simulink model "soc_WLAN_fpga"  (R2024b)
settings: Solver=FixedStepDiscrete  StartTime=0.0  StopTime=stopTime  RelTol=1e-3
PreLoadFcn:
  | addpath(fullfile(matlabroot,'toolbox','whdl','whdlexamples','whdlexamples'));
InitFcn:
  | addpath(fullfile(matlabroot,'toolbox','whdl','whdlexamples','whdlexamples'));
model workspace (MAT data in the model file):
  socvcb : containers.Map (value not decoded)
undefined symbols (not defined in the file): Add, bitRatePerOfdmSym, chanBW, coe, cpLen, dataUpsampleFactor, DelayValMaxNsdMinusLastPilotSc, DescramblerInitialSeed, designMultirateFIR, fftLen, filterLatency, filterUpsampleFactor, Fs, Hd, HT_MFMCS0, HT_MFMCS1, HT_MFMCS2, HT_MFMCS3, HT_MFMCS4, HT_MFMCS5, HT_MFMCS6, HT_MFMCS7, HTUnUsedScInd, inputSamplingRate, interp_coeff, maxPilotRefCounterVale, maxPilotsRef, maxPilotsRefNonHT, Ncol_HT, Ncol_NonHT, noDataSubCarriers, Non_HTMCS0, Non_HTMCS1, Non_HTMCS2, Non_HTMCS3, Non_HTMCS4, Non_HTMCS5, Non_HTMCS6, Non_HTMCS7, Nrow_HT, Nrow_NonHT, numDSC_HT, numDSC_HT_vhtSigB, numDSC_NonHT, numDscHT, numDscNonHT, numOfBitsPerOFDMSym, numOfDataBitsPerOFDMSym, numPilots, numScHT, numSCS_HT, numSCS_NonHT, pnSeq, QAM, rxDownsampleFactor, secondPIdx_HT, secondPIdx_NonHT, Shift, VHTMCS0, VHTMCS1 ... (+7)
libraries: hdlsllib x267, simulink x210, dspsigops x22, whdlutilities x10, whdlmod x9, dsphdlfiltering2 x5, dsphdlmathfun2 x4, whdledac x3, hwlogicconnlib x2, commhdlcrc x2, dsphdlsigops2 x2
(part 3 of 14)

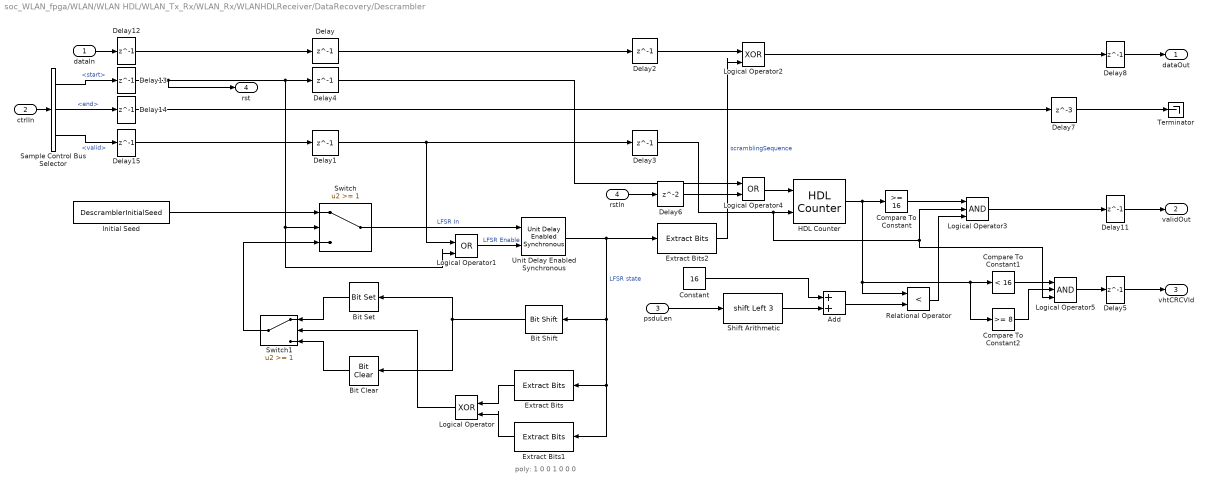
== system soc_WLAN_fpga/WLAN/WLAN HDL/WLAN_Tx_Rx/WLAN_Rx/WLANHDLReceiver/DataRecovery/Descrambler ==
  note: poly: 1 0 0 1 0 0 0
  dataIn : Inport
  ctrlIn : Inport  Port=2
  psduLen : Inport  Port=3
  rstIn : Inport  Port=4
  Add : Sum
  Bit Clear : simulink/Logic and Bit Operations/Bit Clear  iBit=0
  Bit Set : simulink/Logic and Bit Operations/Bit Set  iBit=0
  Bit Shift : hdlsllib/Logic and Bit Operations/Bit Shift  mode=Shift Left Logical  N=1
  Compare To Constant : simulink/Logic and Bit Operations/Compare To Constant  relop=>=  const=16  OutDataTypeStr=boolean
  Compare To Constant1 : simulink/Logic and Bit Operations/Compare To Constant  relop=<  const=16  OutDataTypeStr=boolean
  Compare To Constant2 : simulink/Logic and Bit Operations/Compare To Constant  relop=>=  const=8  OutDataTypeStr=boolean
  Constant : Constant  Value=16  OutDataTypeStr=fixdt(0,5,0)  SampleTime=-1
  Delay{,1..4} (5 alike) : Delay  DelayLength=1
  Delay{5,8,11..15} (7 alike) : Delay  DelayLength=1  InitialCondition=0
  Delay6 : Delay
  Delay7 : Delay  DelayLength=3
  Extract Bits : simulink/Logic and Bit Operations/Extract Bits  bitsToExtract=Range of bits  numBits=8  bitIdxRange=3  outScalingMode=Preserve fixed-point scaling
  Extract Bits1 : simulink/Logic and Bit Operations/Extract Bits  bitsToExtract=Range of bits  numBits=8  bitIdxRange=6  outScalingMode=Preserve fixed-point scaling
  Extract Bits2 : simulink/Logic and Bit Operations/Extract Bits  bitsToExtract=Range of bits  numBits=8  bitIdxRange=0  outScalingMode=Preserve fixed-point scaling
  HDL Counter : hdlsllib/Sources/HDL Counter  CountType=Count limited  CountInit=0  CountStep=1  CountMax=2^32-1  CountFromType=Initial value  CountFrom=0  CountResetPort=on  CountLoadPort=off  CountEnbPort=on  CountDirPort=off  CountHitOutputPort=off  CountDataType=Unsigned  CountWordLen=32  CountFracLen=0  CountSampTime=1
  Initial Seed : Constant  Value=DescramblerInitialSeed  OutDataTypeStr=fixdt(0,7,0)  SampleTime=-1
  Logical Operator : Logic  Operator=XOR  IconShape=distinctive  AllPortsSameDT=off  OutDataTypeStr=boolean
  Logical Operator1 : Logic  Operator=OR  IconShape=distinctive  AllPortsSameDT=off  OutDataTypeStr=boolean
  Logical Operator2 : Logic  Operator=XOR  IconShape=distinctive  AllPortsSameDT=off  OutDataTypeStr=boolean
  Logical Operator3 : Logic  Inputs=3  AllPortsSameDT=off  OutDataTypeStr=boolean
  Logical Operator4 : Logic  Operator=OR  AllPortsSameDT=off  OutDataTypeStr=boolean
  Logical Operator5 : Logic  Inputs=3  AllPortsSameDT=off  OutDataTypeStr=boolean
  Relational Operator : RelationalOperator  Operator=<  OutDataTypeStr=boolean  RndMeth=Simplest  InputSameDT=off
  Sample Control Bus Selector : whdlutilities/Sample Control Bus Selector  OutputSignals=start,end,valid
  Shift Arithmetic : ArithShift  BitShiftNumber=3  BitShiftDirection=Left
  Switch : Switch  Threshold=1  SaturateOnIntegerOverflow=off  InputSameDT=off
  Switch1 : Switch  Threshold=1  SaturateOnIntegerOverflow=off  InputSameDT=off
  Terminator : Terminator
  Unit Delay Enabled Synchronous : hdlsllib/Discrete/Unit Delay Enabled Synchronous  InitialCondition=0.0  SampleTime=-1
  dataOut : Outport
  validOut : Outport  Port=2
  vhtCRCVld : Outport  Port=3
  rst : Outport  Port=4
  wires:
  Delay15/1 -> Delay1/1
  Delay13/1 -> rst/1, Delay4/1, Switch/2, Logical Operator1/2
  Delay12/1 -> Delay/1
  Delay8/1 -> dataOut/1
  Delay4/1 -> Logical Operator4/1
  Delay2/1 -> Logical Operator2/1
  Logical Operator2/1 -> Delay8/1
  Delay1/1 -> Delay3/1, Logical Operator1/1
  Delay/1 -> Delay2/1
  Logical Operator1/1 -> Unit Delay Enabled Synchronous/2  "LFSR Enable"
  Switch1/1 -> Switch/3
  Bit Shift/1 -> Bit Set/1, Bit Clear/1
  Logical Operator/1 -> Switch1/2
  Bit Clear/1 -> Switch1/3
  Bit Set/1 -> Switch1/1
  Extract Bits1/1 -> Logical Operator/2
  Extract Bits/1 -> Logical Operator/1
  Extract Bits2/1 -> Logical Operator2/2  "scramblingSequence"
  dataIn/1 -> Delay12/1
  Unit Delay Enabled Synchronous/1 -> Extract Bits2/1, Extract Bits/1, Extract Bits1/1, Bit Shift/1  "LFSR state"
  Initial Seed/1 -> Switch/1
  Switch/1 -> Unit Delay Enabled Synchronous/1  "LFSR In"
  ctrlIn/1 -> Sample Control Bus Selector/1
  HDL Counter/1 -> Compare To Constant/1, Compare To Constant2/1, Compare To Constant1/1, Relational Operator/1
  Compare To Constant/1 -> Logical Operator3/1
  Shift Arithmetic/1 -> Add/2
  Constant/1 -> Add/1
  Relational Operator/1 -> Logical Operator3/3
  Logical Operator4/1 -> HDL Counter/1
  rstIn/1 -> Delay6/1
  Delay6/1 -> Logical Operator4/2
  Sample Control Bus Selector/1 -> Delay13/1  "<start>"
  Sample Control Bus Selector/2 -> Delay14/1  "<end>"
  Sample Control Bus Selector/3 -> Delay15/1  "<valid>"
  Delay11/1 -> validOut/1
  Compare To Constant1/1 -> Logical Operator5/1
  Compare To Constant2/1 -> Logical Operator5/2
  Delay5/1 -> vhtCRCVld/1
  Delay7/1 -> Terminator/1
  Delay14/1 -> Delay7/1
  Delay3/1 -> Logical Operator5/3, Logical Operator3/2, HDL Counter/2
  Add/1 -> Relational Operator/2
  Logical Operator3/1 -> Delay11/1
  Logical Operator5/1 -> Delay5/1
  psduLen/1 -> Shift Arithmetic/1

== system soc_WLAN_fpga/WLAN/WLAN HDL/WLAN_Tx_Rx/WLAN_Rx/WLANHDLReceiver/DataRecovery/VHT SignalB CRC Check ==
  vhtSigCRCBit : Inport
  vhtSigCRCVld : Inport  Port=2
  vhtCRCRefBit : Inport  Port=3
  vhtCRCRefBitVld : Inport  Port=4
  rstIn : Inport  Port=5
  format : Inport  Port=6
  Compare To Constant : simulink/Logic and Bit Operations/Compare To Constant  relop===  const=2  OutDataTypeStr=boolean
  Delay : Delay  DelayLength=1
  Delay1 : Delay  DelayLength=1
  Delay2 : Delay  DelayLength=1  ExternalReset=Level
      settings: InputPortMap=u0,r5
  HDL Counter : hdlsllib/Sources/HDL Counter  CountType=Count limited  CountInit=0  CountStep=1  CountMax=7  CountFromType=Initial value  CountFrom=0  CountResetPort=on  CountLoadPort=off  CountEnbPort=on  CountDirPort=off  CountHitOutputPort=off  CountDataType=Unsigned  CountWordLen=3  CountFracLen=0  CountSampTime=1
  HDL Counter1 : hdlsllib/Sources/HDL Counter  CountType=Count limited  CountInit=0  CountStep=1  CountMax=7  CountFromType=Initial value  CountFrom=0  CountResetPort=on  CountLoadPort=off  CountEnbPort=on  CountDirPort=off  CountHitOutputPort=off  CountDataType=Unsigned  CountWordLen=3  CountFracLen=0  CountSampTime=1
  Logical Operator : Logic  Inputs=3  AllPortsSameDT=off  OutDataTypeStr=boolean
  Logical Operator1 : Logic  Operator=OR  AllPortsSameDT=off  OutDataTypeStr=boolean
  Relational Operator : RelationalOperator  Operator=~=  OutDataTypeStr=boolean  RndMeth=Simplest  InputSameDT=off
  Simple Dual Port RAM : hdlsllib/HDL RAMs/Simple Dual Port RAM  ram_size=3
  VHTSigCRCStatus : Outport
  wires:
  HDL Counter/1 -> Simple Dual Port RAM/2
  vhtCRCRefBit/1 -> Simple Dual Port RAM/1
  vhtCRCRefBitVld/1 -> HDL Counter/2, Simple Dual Port RAM/3
  vhtSigCRCVld/1 -> Delay1/1, HDL Counter1/2
  HDL Counter1/1 -> Simple Dual Port RAM/4
  vhtSigCRCBit/1 -> Delay/1
  Simple Dual Port RAM/1 -> Relational Operator/1
  Delay/1 -> Relational Operator/2
  Logical Operator/1 -> Logical Operator1/1
  rstIn/1 -> HDL Counter/1, Delay2/2, HDL Counter1/1
  Relational Operator/1 -> Logical Operator/1
  Delay1/1 -> Logical Operator/2
  Logical Operator1/1 -> VHTSigCRCStatus/1, Delay2/1
  Delay2/1 -> Logical Operator1/2
  format/1 -> Compare To Constant/1
  Compare To Constant/1 -> Logical Operator/3

== system soc_WLAN_fpga/WLAN/WLAN HDL/WLAN_Tx_Rx/WLAN_Rx/WLANHDLReceiver/DataRecovery/VHTSigBMCS ==
  note: Selecting BPSK and 1/2 rate coding for VHT Signal B field
  enb : Inport
  modSel : Inport  Port=2
  codeRate : Inport  Port=3
  format : Inport  Port=4
  rst : Inport  Port=5
  Compare To Constant : simulink/Logic and Bit Operations/Compare To Constant  relop=<=  const=numDSC_HT-1  OutDataTypeStr=boolean
  Compare To Constant1 : simulink/Logic and Bit Operations/Compare To Constant  relop===  const=2  OutDataTypeStr=boolean
  Constant : Constant  Value=fi(0,0,3,0)  SampleTime=-1
  Constant1 : Constant  Value=fi(0,0,2,0)  SampleTime=-1
  HDL Counter : hdlsllib/Sources/HDL Counter  CountType=Count limited  CountInit=0  CountStep=1  CountMax=65535  CountFromType=Initial value  CountFrom=0  CountResetPort=on  CountLoadPort=off  CountEnbPort=on  CountDirPort=off  CountHitOutputPort=off  CountDataType=Unsigned  CountWordLen=16  CountFracLen=0  CountSampTime=1
  Logical Operator : Logic  AllPortsSameDT=off  OutDataTypeStr=boolean
  Switch : Switch  Criteria=u2 ~= 0  SaturateOnIntegerOverflow=off  InputSameDT=off
  Switch1 : Switch  Criteria=u2 ~= 0  SaturateOnIntegerOverflow=off  InputSameDT=off
  modSelOut : Outport
  codeRateOut : Outport  Port=2
  wires:
  modSel/1 -> Switch/3
  Compare To Constant/1 -> Logical Operator/1
  Switch/1 -> modSelOut/1
  Compare To Constant1/1 -> Logical Operator/2
  HDL Counter/1 -> Compare To Constant/1
  Logical Operator/1 -> Switch1/2, Switch/2
  Constant/1 -> Switch/1
  enb/1 -> HDL Counter/2
  format/1 -> Compare To Constant1/1
  rst/1 -> HDL Counter/1
  codeRate/1 -> Switch1/3
  Constant1/1 -> Switch1/1
  Switch1/1 -> codeRateOut/1

== system soc_WLAN_fpga/WLAN/WLAN HDL/WLAN_Tx_Rx/WLAN_Rx/WLANHDLReceiver/DataRecovery/rateMapping ==
  note: decoderInpLen = ceil((psduLen+22)/(numSCs*modOrder*codeRate))*(numSCs*modOrder)
  note: codeRate
  note: modSel
  note: numSCs*modOrder
  note: 1/(numSCs*modOrder*codeRate)
  MCS : Inport
  frameFormat : Inport  Port=2
  psduLen : Inport  Port=3
  1-D Lookup Table : Lookup_n-D  BreakpointsForDimension1=[0:3]  BreakpointsForDimension2=[0:7]  IndexSearchMethod=Evenly spaced points  Table=[48*[1,1,2,2,4,4,6,6];52*[1,2,2,4,4,6,6,6];52*[1,2,2,4,4,6,6,6];52*[1,2,2,4,4,6,6,6]]  TableDataTypeStr=fixdt(0,16,0)  ExtrapMethod=Clip  UseLastTableValue=on  InternalRulePriority=Speed  OutDataTypeStr=fixdt(0,16,0)  RndMeth=Simplest
      settings: InputPortMap=u0,u1
  1-D Lookup Table1 : Lookup_n-D  BreakpointsForDimension1=[0:3]  BreakpointsForDimension2=[0:7]  IndexSearchMethod=Evenly spaced points  Table=fi(1./[24,36,48,72,96,144,192,216;26,52,78,104,156,208,234,260;26,52,78,104,156,208,234,260;26,52,78,104,156,208,234,260],0,16,16)  TableDataTypeStr=fixdt(0,16,16)  ExtrapMethod=Clip  UseLastTableValue=on  InternalRulePriority=Speed  OutDataTypeStr=fixdt(0,16,16)  RndMeth=Simplest
      settings: InputPortMap=u0,u1
  1-D Lookup Table2 : Lookup_n-D  BreakpointsForDimension1=[0:3]  BreakpointsForDimension2=[0:7]  IndexSearchMethod=Evenly spaced points  Table=[0,0,1,1,4,4,6,6;0,1,1,4,4,6,6,6;0,1,1,4,4,6,6,6;0,1,1,4,4,6,6,6]  TableDataTypeStr=fixdt(0,3,0)  ExtrapMethod=Clip  UseLastTableValue=on  InternalRulePriority=Speed  OutDataTypeStr=fixdt(0,3,0)  RndMeth=Simplest
      settings: InputPortMap=u0,u1
  1-D Lookup Table3 : Lookup_n-D  BreakpointsForDimension1=[0:3]  BreakpointsForDimension2=[0:7]  IndexSearchMethod=Evenly spaced points  Table=[0,2,0,2,0,2,1,2;0,0,2,0,2,1,2,3;0,0,2,0,2,1,2,3;0,0,2,0,2,1,2,3]  TableDataTypeStr=fixdt(0,2,0)  ExtrapMethod=Clip  UseLastTableValue=on  InternalRulePriority=Speed  OutDataTypeStr=fixdt(0,2,0)  RndMeth=Simplest
      settings: InputPortMap=u0,u1
  Add : Sum
  Constant1 : Constant  Value=fi(22,0,5,0)  SampleTime=-1
  Data Type Conversion : DataTypeConversion  OutDataTypeStr=uint16  RndMeth=Ceiling  SaturateOnIntegerOverflow=off
  Data Type Conversion : DataTypeConversion  OutDataTypeStr=fixdt(0,3,0)  SaturateOnIntegerOverflow=off  RndMeth=Floor
  Delay{,1..5,11} (7 alike) : Delay  DelayLength=1
  Delay{6..10} (5 alike) : Delay
  Delay12 : Delay  DelayLength=6
  Delay13 : Delay  DelayLength=6
  Product1 : Product  OutDataTypeStr=fixdt(0,17,0)  RndMeth=Ceiling
  Product4 : Product  RndMeth=Ceiling  OutDataTypeStr=Inherit: Same as first input
  Shift Arithmetic : ArithShift  BitShiftNumber=3  BitShiftDirection=Left
  modSel : Outport
  codeRate : Outport  Port=2
  decoderInpLen : Outport  Port=3
  wires:
  frameFormat/1 -> Delay1/1
  1-D Lookup Table1/1 -> Delay5/1
  1-D Lookup Table/1 -> Delay4/1
  Data Type Conversion/1 -> Product1/1  "numSymbols"
  Product4/1 -> Delay9/1
  Add/1 -> Delay6/1
  Constant1/1 -> Add/2
  Shift Arithmetic/1 -> Delay3/1
  psduLen/1 -> Delay/1
  MCS/1 -> Delay2/1
  Product1/1 -> Delay11/1
  1-D Lookup Table2/1 -> Delay12/1
  1-D Lookup Table3/1 -> Delay13/1
  Data Type Conversion/1 -> 1-D Lookup Table3/1, 1-D Lookup Table2/1, 1-D Lookup Table1/1, 1-D Lookup Table/1
  Delay/1 -> Shift Arithmetic/1
  Delay1/1 -> Data Type Conversion/1
  Delay2/1 -> 1-D Lookup Table/2, 1-D Lookup Table1/2, 1-D Lookup Table2/2, 1-D Lookup Table3/2
  Delay3/1 -> Add/1
  Delay4/1 -> Delay8/1
  Delay5/1 -> Delay7/1
  Delay6/1 -> Product4/1
  Delay7/1 -> Product4/2
  Delay8/1 -> Delay10/1
  Delay9/1 -> Data Type Conversion/1
  Delay10/1 -> Product1/2
  Delay11/1 -> decoderInpLen/1
  Delay12/1 -> modSel/1
  Delay13/1 -> codeRate/1

== system soc_WLAN_fpga/WLAN/WLAN HDL/WLAN_Tx_Rx/WLAN_Rx/WLANHDLReceiver/DataRecovery/symbolDemodulator ==
  dataIn : Inport
  validIn : Inport  Port=2
  modSel : Inport  Port=3
  codeRate : Inport  Port=4
  numSCs : Inport  Port=5
  rstIn : Inport  Port=6
  Compare To Constant : simulink/Logic and Bit Operations/Compare To Constant  relop===  const=0  OutDataTypeStr=boolean
  Compare To Constant2 : simulink/Logic and Bit Operations/Compare To Constant  relop===  const=1  OutDataTypeStr=boolean
  Constant : Constant  Value=fi(1,0,1,0)  SampleTime=-1
  Delay1 : Delay  DelayLength=7
  Delay2 : Delay  DelayLength=7
  Delay{3..6} (4 alike) : Delay  DelayLength=15
  Gain : Gain  Gain=-1  OutDataTypeStr=Inherit: Same as input
  Gain2 : Gain  Gain=-1  OutDataTypeStr=Inherit: Same as input
  HDL Counter : hdlsllib/Sources/HDL Counter  CountType=Count limited  CountInit=0  CountStep=1  CountMax=numDSC_HT-1  CountFromType=Initial value  CountFrom=0  CountResetPort=on  CountLoadPort=off  CountEnbPort=on  CountDirPort=off  CountHitOutputPort=off  CountDataType=Unsigned  CountWordLen=8  CountFracLen=0  CountSampTime=1
  HDL Counter1 : hdlsllib/Sources/HDL Counter  CountType=Count limited  CountInit=0  CountStep=1  CountMax=1  CountFromType=Initial value  CountFrom=0  CountResetPort=on  CountLoadPort=off  CountEnbPort=on  CountDirPort=off  CountHitOutputPort=off  CountDataType=Unsigned  CountWordLen=8  CountFracLen=0  CountSampTime=1
  Logical Operator : Logic  Operator=OR  AllPortsSameDT=off  OutDataTypeStr=boolean
  Logical Operator1 : Logic  AllPortsSameDT=off  OutDataTypeStr=boolean
  Logical Operator2 : Logic  AllPortsSameDT=off  OutDataTypeStr=boolean
  Relational Operator : RelationalOperator  Operator===  OutDataTypeStr=boolean  RndMeth=Simplest  InputSameDT=off
  Subtract : Sum  Inputs=+-
  Switch : Switch  Criteria=u2 ~= 0  SaturateOnIntegerOverflow=off  InputSameDT=off
  Switch2 : Switch  Criteria=u2 ~= 0  SaturateOnIntegerOverflow=off  InputSameDT=off
  Switch3 : Switch  Criteria=u2 ~= 0  SaturateOnIntegerOverflow=off  InputSameDT=off
  Symbol Demodulator : whdlmod/Symbol Demodulator  ModulationSource=Input port  ModulationScheme=BPSK  MaxModulation=64-QAM  ConstOrder=Default  ConstMap=[ 2, 3, 1, 0, 6, 7, 5, 4, 14, 15, 13, 12, 10, 11, 9, 8 ]  DecisionType=Approximate log-likelihood ratio  PhaseOffset=0  OutputType=Scalar  NormMethod=Unit average power  MinSymDistance=2  NoiseVariance=off  SimulateUsing=Code generation
  Symbol Demodulator1 : whdlmod/Symbol Demodulator  ModulationSource=Input port  ModulationScheme=QPSK  MaxModulation=QPSK  ConstOrder=User-defined  ConstMap=[ 2, 3, 1, 0, 6, 7, 5, 4, 14, 15, 13, 12, 10, 11, 9, 8 ]  DecisionType=Approximate log-likelihood ratio  PhaseOffset=-pi/4  OutputType=Scalar  NormMethod=Unit average power  MinSymDistance=2  NoiseVariance=off  SimulateUsing=Code generation
  Terminator1 : Terminator
  Terminator5 : Terminator
  sampleAndHold : MATLAB Function  TreatAsAtomicUnit=on
  dataOut : Outport
  validOut : Outport  Port=2
  numSCsOut : Outport  Port=3
  modSelOut : Outport  Port=4
  codeRateOut : Outport  Port=5
  rstOut : Outport  Port=6
  wires:
  Logical Operator/1 -> HDL Counter/1
  Compare To Constant/1 -> Logical Operator1/1
  sampleAndHold/2(codeRateOut) -> Delay5/1
  Logical Operator1/1 -> sampleAndHold/3(enb)
  Subtract/1 -> Delay4/1, Relational Operator/2
  Logical Operator2/1 -> Logical Operator/1
  Delay6/1 -> rstOut/1
  codeRate/1 -> sampleAndHold/2(codeRateIn)
  Symbol Demodulator/2 -> validOut/1
  Delay5/1 -> codeRateOut/1
  Symbol Demodulator/3 -> Terminator5/1
  modSel/1 -> sampleAndHold/1(modSelIn)
  Delay3/1 -> modSelOut/1
  Relational Operator/1 -> Logical Operator2/1
  Delay4/1 -> numSCsOut/1
  sampleAndHold/1(modSelOut) -> Switch/2, Symbol Demodulator1/3, Symbol Demodulator/3, Compare To Constant2/1, Delay3/1
  rstIn/1 -> Delay6/1, HDL Counter1/1, sampleAndHold/4(reset), Logical Operator/2
  HDL Counter/1 -> Compare To Constant/1, Relational Operator/1
  dataIn/1 -> Symbol Demodulator1/1, Symbol Demodulator/1
  numSCs/1 -> Subtract/1
  Constant/1 -> Subtract/2
  validIn/1 -> Symbol Demodulator1/2, Symbol Demodulator/2, Logical Operator2/2, Logical Operator1/2, HDL Counter/2
  Symbol Demodulator/1 -> Gain/1, Switch/1
  Switch/1 -> Switch3/3
  Gain/1 -> Switch/3
  Symbol Demodulator1/1 -> Delay1/1
  Symbol Demodulator1/2 -> Delay2/1
  Symbol Demodulator1/3 -> Terminator1/1
  Delay2/1 -> HDL Counter1/2
  HDL Counter1/1 -> Switch2/2
  Delay1/1 -> Gain2/1, Switch2/1
  Gain2/1 -> Switch2/3
  Compare To Constant2/1 -> Switch3/2
  Switch2/1 -> Switch3/1
  Switch3/1 -> dataOut/1

== system soc_WLAN_fpga/WLAN/WLAN HDL/WLAN_Tx_Rx/WLAN_Rx/WLANHDLReceiver/FrameFormatDetectionAndSignalRecovery/CRCCheckAndBitInterpretation ==
  note: Choose bits from 25 to end for VHT Sig parameters
  note: Choose bits from 25 to 65 for CRC detection
  bit : Inport
  <valid> : Inport  Port=2
  formatDetected : Inport  Port=3
  rst : Inport  Port=4
  Compare To Constant : simulink/Logic and Bit Operations/Compare To Constant  relop===  const=1  OutDataTypeStr=boolean
  Compare To Constant1 : simulink/Logic and Bit Operations/Compare To Constant  relop===  const=24  OutDataTypeStr=boolean
  Compare To Constant2 : simulink/Logic and Bit Operations/Compare To Constant  relop=>=  const=24  OutDataTypeStr=boolean
  Compare To Constant3 : simulink/Logic and Bit Operations/Compare To Constant  relop===  const=24+42-1  OutDataTypeStr=boolean
  Compare To Constant4 : simulink/Logic and Bit Operations/Compare To Constant  relop=<=  const=24+42-1  OutDataTypeStr=boolean
  Compare To Constant6 : simulink/Logic and Bit Operations/Compare To Constant  relop=>=  const=24  OutDataTypeStr=boolean
  Data Type Conversion : DataTypeConversion  OutDataTypeStr=fixdt(0,3,0)  SaturateOnIntegerOverflow=off  RndMeth=Floor
  Delay : Delay  DelayLength=5*(cpLen+fftLen)
  General CRC Syndrome Detector HDL Optimized : commhdlcrc/General CRC Syndrome Detector HDL Optimized  Polynomial=[1 0 0 0 0 0 1 1 1]  InitialState=1  DirectMethod=on  ReflectInput=off  ReflectCRCChecksum=off  FinalXORValue=1  SimulateUsing=Code generation
  HDL Counter : hdlsllib/Sources/HDL Counter  CountType=Count limited  CountInit=0  CountStep=1  CountMax=71  CountFromType=Initial value  CountFrom=0  CountResetPort=on  CountLoadPort=off  CountEnbPort=on  CountDirPort=off  CountHitOutputPort=off  CountDataType=Unsigned  CountWordLen=8  CountFracLen=0  CountSampTime=1
  HDL Counter1 : hdlsllib/Sources/HDL Counter  CountType=Count limited  CountInit=0  CountStep=1  CountMax=71  CountFromType=Initial value  CountFrom=0  CountResetPort=on  CountLoadPort=off  CountEnbPort=on  CountDirPort=off  CountHitOutputPort=off  CountDataType=Unsigned  CountWordLen=8  CountFracLen=0  CountSampTime=1
  HTSigBitRecover : MATLAB Function  TreatAsAtomicUnit=on
  LSigBitRecover : MATLAB Function  TreatAsAtomicUnit=on
  Logical Operator{,1..3} (4 alike) : Logic  AllPortsSameDT=off  OutDataTypeStr=boolean
  Multiport Switch : MultiPortSwitch  DataPortOrder=Zero-based contiguous  zeroidx=on  SaturateOnIntegerOverflow=off  InputSameDT=off
  Repeat3 : dspsigops/Repeat  FactorSource=Dialog parameter  N=dataUpsampleFactor  Nmax=16  RateOptions=Allow multirate processing  ic=0  mode=Unused parameter value
  Switch1 : Switch  Criteria=u2 > Threshold  SaturateOnIntegerOverflow=off  InputSameDT=off
  Terminator{,1..3} (4 alike) : Terminator
  VHTSigBitRecover : MATLAB Function  TreatAsAtomicUnit=on
  numOFDMSymbolCalVHT : Subsystem
  failCheck : Outport
  PSDULen : Outport  Port=2
  HTCRCStatus : Outport  Port=3
  MCS : Outport  Port=4
  numOFDMSymbVHT : Outport  Port=5
  wires:
  LSigBitRecover/2(MCS) -> Multiport Switch/2
  HTSigBitRecover/1(MCS) -> Multiport Switch/3
  HTSigBitRecover/2(PSDULen) -> Switch1/1
  HDL Counter/1 -> Compare To Constant4/1, Compare To Constant3/1, Compare To Constant1/1, Compare To Constant2/1
  Compare To Constant2/1 -> Logical Operator/2
  Compare To Constant1/1 -> General CRC Syndrome Detector HDL Optimized/2
  Compare To Constant3/1 -> General CRC Syndrome Detector HDL Optimized/3
  Logical Operator1/1 -> General CRC Syndrome Detector HDL Optimized/4
  Logical Operator/1 -> HTSigBitRecover/2(validIn), Logical Operator1/1
  Compare To Constant4/1 -> Logical Operator1/2
  General CRC Syndrome Detector HDL Optimized/1 -> Terminator/1
  General CRC Syndrome Detector HDL Optimized/2 -> Terminator1/1
  General CRC Syndrome Detector HDL Optimized/3 -> Terminator2/1
  General CRC Syndrome Detector HDL Optimized/4 -> Terminator3/1
  General CRC Syndrome Detector HDL Optimized/5 -> Logical Operator2/1
  formatDetected/1 -> Switch1/2, Compare To Constant/1, Multiport Switch/1
  Multiport Switch/1 -> Data Type Conversion/1
  LSigBitRecover/3(PSDULen) -> numOFDMSymbolCalVHT/1(PSDULenNonHT), Switch1/3
  Switch1/1 -> PSDULen/1
  LSigBitRecover/1(failCheck) -> failCheck/1
  <valid>/1 -> LSigBitRecover/2(validIn), Logical Operator/1, Logical Operator3/1, HDL Counter1/2, HDL Counter/2
  Compare To Constant6/1 -> Logical Operator3/2
  Logical Operator3/1 -> VHTSigBitRecover/2(validIn)
  HDL Counter1/1 -> Compare To Constant6/1
  VHTSigBitRecover/1(MCS) -> Multiport Switch/4
  bit/1 -> HTSigBitRecover/1(bit), VHTSigBitRecover/1(bit), General CRC Syndrome Detector HDL Optimized/1, LSigBitRecover/1(bit)
  Data Type Conversion/1 -> MCS/1
  Repeat3/1 -> HTCRCStatus/1  "signalCRCStatus"
  Compare To Constant/1 -> Logical Operator2/2
  Logical Operator2/1 -> Repeat3/1
  rst/1 -> HTSigBitRecover/3(rst), VHTSigBitRecover/3(rst), Delay/1, HDL Counter1/1, HDL Counter/1
  Delay/1 -> LSigBitRecover/3(rst)
  VHTSigBitRecover/2(numSTS) -> numOFDMSymbolCalVHT/2(numSTS)
  numOFDMSymbolCalVHT/1(numOFDMSymbVHT) -> numOFDMSymbVHT/1

== system soc_WLAN_fpga/WLAN/WLAN HDL/WLAN_Tx_Rx/WLAN_Rx/WLANHDLReceiver/FrameFormatDetectionAndSignalRecovery/FormatIdentification ==
  note: Delays to match arrival of MCS
  dataIn : Inport
  validIn : Inport  Port=2
  symbCount : Inport  Port=3
  rst : Inport  Port=4
  MCS : Inport  Port=5
  Compare To Zero : simulink/Logic and Bit Operations/Compare To Zero  relop===  OutDataTypeStr=boolean
  Delay : Delay  DelayLength=3
  Delay1 : Delay  DelayLength=197
  Delay2 : Delay  DelayLength=197
  Delay3 : Delay  DelayLength=197
  Delay4 : Delay  DelayLength=3
  Delay5 : Delay  DelayLength=3
  HDL Counter : hdlsllib/Sources/HDL Counter  CountType=Count limited  CountInit=0  CountStep=1  CountMax=65535  CountFromType=Initial value  CountFrom=0  CountResetPort=on  CountLoadPort=off  CountEnbPort=on  CountDirPort=off  CountHitOutputPort=off  CountDataType=Unsigned  CountWordLen=16  CountFracLen=0  CountSampTime=1
  Logical Operator : Logic  AllPortsSameDT=off  OutDataTypeStr=boolean
  frameFormatMapping : MATLAB Function  TreatAsAtomicUnit=on
  isQBPSK : Subsystem
  formatDetected : Outport
  frameFormat : Outport  Port=2
  wires:
  dataIn/1 -> isQBPSK/1(dataIn)
  isQBPSK/1(isQBPSK) -> Delay1/1
  validIn/1 -> isQBPSK/2(validIn)
  symbCount/1 -> isQBPSK/3(symbCount), Delay5/1
  MCS/1 -> Delay/1
  frameFormatMapping/1(frameFormat) -> frameFormat/1
  frameFormatMapping/2(formatDetected) -> Logical Operator/2, HDL Counter/2
  HDL Counter/1 -> Compare To Zero/1
  Compare To Zero/1 -> Logical Operator/1
  Logical Operator/1 -> formatDetected/1
  Delay1/1 -> frameFormatMapping/3(isQBPSK)
  Delay2/1 -> frameFormatMapping/1(symbNum)
  Delay/1 -> frameFormatMapping/2(MCS)
  rst/1 -> Delay4/1, isQBPSK/4(rst)
  Delay3/1 -> HDL Counter/1, frameFormatMapping/4(reset)
  Delay4/1 -> Delay3/1
  Delay5/1 -> Delay2/1

== system soc_WLAN_fpga/WLAN/WLAN HDL/WLAN_Tx_Rx/WLAN_Rx/WLANHDLReceiver/FrameFormatDetectionAndSignalRecovery/SignalBitRecovery ==
  dataIn : Inport
  dataSCValid : Inport  Port=2
  modSel : Inport  Port=3
  rst : Inport  Port=4
  numSCS : Inport  Port=5
  Bus Creator : BusCreator  Inputs=2  OutDataTypeStr=Bus: hconstellationBus  NonVirtualBus=on
  Compare To Constant : simulink/Logic and Bit Operations/Compare To Constant  relop===  const=0  OutDataTypeStr=boolean
  Data Type Conversion : DataTypeConversion  OutDataTypeStr=int8  SaturateOnIntegerOverflow=off  RndMeth=Floor
  Deinterleaver Block : Subsystem  mask{isInterleaver=off, maxBlkSize=48, nColumns=16}
      mask prompts: isInterleaver "Interleaver"; maxBlkSize "Maximum block size:"; nColumns "Number of columns:"
      mask init:
      | maxNRows = maxBlkSize/nColumns;
      mask DialogControl ParameterGroupVar Prompt: Interleaver/Deinterleaver
      mask DialogControl Control1 Prompt: Select the Interleaver parameter to use the block as an Interleaver and clear the parameter to use the block as a Deinterleaver.
  Delay : Delay  DelayLength=13
  Delay1 : Delay  DelayLength=5
  Delay2 : Delay  DelayLength=5
  Gain : Gain  Gain=-1  OutDataTypeStr=Inherit: Same as input
  HDL Counter1 : hdlsllib/Sources/HDL Counter  CountType=Count limited  CountInit=0  CountStep=1  CountMax=numDSC_NonHT-1  CountFromType=Initial value  CountFrom=0  CountResetPort=on  CountLoadPort=off  CountEnbPort=on  CountDirPort=off  CountHitOutputPort=off  CountDataType=Unsigned  CountWordLen=8  CountFracLen=0  CountSampTime=1
  Logical Operator : Logic  AllPortsSameDT=off  OutDataTypeStr=boolean
  Logical Operator1 : Logic  AllPortsSameDT=off  OutDataTypeStr=boolean
  Logical Operator2 : Logic  Operator=OR  AllPortsSameDT=off  OutDataTypeStr=boolean
  Relational Operator : RelationalOperator  Operator===  OutDataTypeStr=boolean  RndMeth=Simplest  InputSameDT=off
  Repeat1 : dspsigops/Repeat  FactorSource=Dialog parameter  N=dataUpsampleFactor  Nmax=16  RateOptions=Allow multirate processing  ic=0  mode=Unused parameter value
  Repeat6 : dspsigops/Repeat  FactorSource=Dialog parameter  N=dataUpsampleFactor  Nmax=16  RateOptions=Allow multirate processing  ic=0  mode=Unused parameter value
  Sample Control Bus Creator : whdlutilities/Sample Control Bus Creator
  Switch : Switch  Criteria=u2 ~= 0  SaturateOnIntegerOverflow=off  InputSameDT=off
  Switch1 : Switch  Criteria=u2 ~= 0  SaturateOnIntegerOverflow=off  InputSameDT=off
  Symbol Demodulator : whdlmod/Symbol Demodulator  ModulationSource=Property  ModulationScheme=BPSK  MaxModulation=256-QAM  ConstOrder=Default  ConstMap=[ 2, 3, 1, 0, 6, 7, 5, 4, 14, 15, 13, 12, 10, 11, 9, 8 ]  DecisionType=Approximate log-likelihood ratio  PhaseOffset=pi/2  OutputType=Scalar  NormMethod=Unit average power  MinSymDistance=2  NoiseVariance=off  SimulateUsing=Code generation
  Symbol Demodulator1 : whdlmod/Symbol Demodulator  ModulationSource=Property  ModulationScheme=BPSK  MaxModulation=256-QAM  ConstOrder=Default  ConstMap=[ 2, 3, 1, 0, 6, 7, 5, 4, 14, 15, 13, 12, 10, 11, 9, 8 ]  DecisionType=Approximate log-likelihood ratio  PhaseOffset=0  OutputType=Scalar  NormMethod=Unit average power  MinSymDistance=2  NoiseVariance=off  SimulateUsing=Code generation
  Terminator{,1,5..7} (5 alike) : Terminator
  ViterbiDecoder : Subsystem
  sampleParallel : MATLAB Function  TreatAsAtomicUnit=on
  signBit : Outport
  ctrlOut : Outport  Port=2
  headerConstellation : Outport  Port=3
  wires:
  Logical Operator/1 -> Deinterleaver Block/2(startIn)
  Deinterleaver Block/5(ready) -> Terminator/1
  sampleParallel/3(endOut) -> Sample Control Bus Creator/2
  Deinterleaver Block/2(startOut) -> Terminator6/1
  Compare To Constant/1 -> Logical Operator/1
  sampleParallel/4(validOut) -> Sample Control Bus Creator/3
  Deinterleaver Block/4(validOut) -> sampleParallel/2(validIn)
  Relational Operator/1 -> Logical Operator2/2, Logical Operator1/2
  Logical Operator1/1 -> Deinterleaver Block/3(endIn)
  Switch/1 -> Gain/1
  sampleParallel/2(startOut) -> Sample Control Bus Creator/1
  Symbol Demodulator/3 -> Terminator5/1
  Deinterleaver Block/1(dataOut) -> sampleParallel/1(dataIn)
  Deinterleaver Block/3(endOut) -> Terminator7/1
  HDL Counter1/1 -> Relational Operator/2, Compare To Constant/1
  Switch1/1 -> Logical Operator1/1, HDL Counter1/2, Deinterleaver Block/4(validIn), Logical Operator/2
  modSel/1 -> Switch/2, Switch1/2
  rst/1 -> Delay1/1, Logical Operator2/1
  Repeat1/1 -> Bus Creator/2  "headerConstellationValid"
  Repeat6/1 -> Bus Creator/1  "headerConstellationPoints"
  Bus Creator/1 -> headerConstellation/1
  dataSCValid/1 -> Symbol Demodulator/2, Symbol Demodulator1/2, Repeat1/1
  sampleParallel/1(dataOut) -> ViterbiDecoder/1(llr)
  Sample Control Bus Creator/1 -> ViterbiDecoder/2(ctrlIn)
  ViterbiDecoder/1(bit) -> signBit/1
  ViterbiDecoder/2(ctrlOut) -> ctrlOut/1
  dataIn/1 -> Symbol Demodulator/1, Symbol Demodulator1/1, Repeat6/1
  numSCS/1 -> Delay/1
  Logical Operator2/1 -> HDL Counter1/1
  Delay/1 -> Relational Operator/1
  Delay1/1 -> Delay2/1
  Delay2/1 -> sampleParallel/3(rst)
  Data Type Conversion/1 -> Deinterleaver Block/1(dataIn)
  Gain/1 -> Data Type Conversion/1
  Symbol Demodulator1/3 -> Terminator1/1
  Symbol Demodulator/1 -> Switch/1
  Symbol Demodulator1/2 -> Switch1/3
  Symbol Demodulator/2 -> Switch1/1
  Symbol Demodulator1/1 -> Switch/3

== system soc_WLAN_fpga/WLAN/WLAN HDL/WLAN_Tx_Rx/WLAN_Rx/WLANHDLReceiver/FrameFormatDetectionAndSignalRecovery/SignalFieldController ==
  note: Choose L-SIG, HT-SIG and VHT-SIG based on format detected
  note: Choose BPSK
  note: choose L Sig
  note: For QBPSK
  note: Choose QBPSK
  dataIn : Inport
  validIn : Inport  Port=2
  rd_dout : Inport  Port=3
  validOut : Inport  Port=4
  symbNum : Inport  Port=5
  rst : Inport  Port=6
  formatDetected : Inport  Port=7
  Compare To Constant : simulink/Logic and Bit Operations/Compare To Constant  relop===  const=4  OutDataTypeStr=boolean
  Constant : Constant  Value=0  OutDataTypeStr=fixdt(0,3,0)  SampleTime=-1
  Constant1 : Constant  Value=5  OutDataTypeStr=fixdt(0,3,0)  SampleTime=-1
  Constant2 : Constant  Value=48  OutDataTypeStr=fixdt(0,9,0)  SampleTime=-1
  Constant3 : Constant  Value=48  OutDataTypeStr=fixdt(0,9,0)  SampleTime=-1
  Constant4 : Constant  Value=fi(1,0,1,0)  SampleTime=-1
  Gain : Gain  Gain=-1i  OutDataTypeStr=Inherit: Same as input
  HDL Counter : hdlsllib/Sources/HDL Counter  CountType=Count limited  CountInit=0  CountStep=1  CountMax=numSCS_NonHT*2 - 1  CountFromType=Initial value  CountFrom=0  CountResetPort=on  CountLoadPort=off  CountEnbPort=on  CountDirPort=off  CountHitOutputPort=off  CountDataType=Unsigned  CountWordLen=8  CountFracLen=0  CountSampTime=1
  Logical Operator : Logic  AllPortsSameDT=off  OutDataTypeStr=boolean
  Subtract : Sum  Inputs=+-
  Switch{1..4} (4 alike) : Switch  Criteria=u2 > Threshold  SaturateOnIntegerOverflow=off  InputSameDT=off
  Switch5 : Switch  Criteria=u2 > Threshold  Threshold=1  SaturateOnIntegerOverflow=off  InputSameDT=off
  Switch6 : Switch  Threshold=48  SaturateOnIntegerOverflow=off  InputSameDT=off
  Switch7 : Switch  Criteria=u2 > Threshold  Threshold=1  SaturateOnIntegerOverflow=off  InputSameDT=off
  dataOut : Outport
  dataSCValid : Outport  Port=2
  modSel : Outport  Port=3
  numSCS : Outport  Port=4
  wires:
  Switch3/1 -> dataOut/1
  Switch1/1 -> dataSCValid/1
  validOut/1 -> HDL Counter/2, Switch1/1
  Switch4/1 -> modSel/1
  Constant/1 -> Switch4/3, Switch5/1
  rd_dout/1 -> Switch6/3, Gain/1, Switch7/3
  Gain/1 -> Switch6/1
  Switch6/1 -> Switch7/1
  HDL Counter/1 -> Switch6/2
  Switch7/1 -> Switch3/1
  Switch5/1 -> Switch4/1
  symbNum/1 -> Compare To Constant/1
  Compare To Constant/1 -> Switch2/2, Logical Operator/2
  Logical Operator/1 -> Switch1/3
  validIn/1 -> Logical Operator/1
  dataIn/1 -> Switch3/3
  Constant1/1 -> Switch5/3
  formatDetected/1 -> Switch7/2, Switch4/2, Switch5/2, Switch1/2, Switch3/2
  rst/1 -> HDL Counter/1
  Switch2/1 -> Subtract/1
  Constant2/1 -> Switch2/1
  Constant3/1 -> Switch2/3
  Subtract/1 -> numSCS/1
  Constant4/1 -> Subtract/2

== system soc_WLAN_fpga/WLAN/WLAN HDL/WLAN_Tx_Rx/WLAN_Rx/WLANHDLReceiver/FrameFormatDetectionAndSignalRecovery/averageSigFieldsFor40MHz ==
  In1 : Inport
  In2 : Inport  Port=2
  rst : Inport  Port=3
  Compare To Constant : simulink/Logic and Bit Operations/Compare To Constant  relop===  const=2  OutDataTypeStr=boolean
  Constant : Constant  Value=chanBW  OutDataTypeStr=fixdt(0,3,0)  SampleTime=-1
  Switch : Switch  Criteria=u2 ~= 0  SaturateOnIntegerOverflow=off  InputSameDT=off
  Switch1 : Switch  Criteria=u2 ~= 0  SaturateOnIntegerOverflow=off  InputSameDT=off
  averager : Subsystem
  Out1 : Outport
  Out2 : Outport  Port=2
  wires:
  averager/1(Out1) -> Switch/1
  averager/2(validIn) -> Switch1/1
  In1/1 -> averager/1(In1), Switch/3
  Switch/1 -> Out1/1
  Constant/1 -> Compare To Constant/1
  Compare To Constant/1 -> Switch/2, Switch1/2
  Switch1/1 -> Out2/1
  In2/1 -> Switch1/3, averager/2(enb)
  rst/1 -> averager/3(rst)

== system soc_WLAN_fpga/WLAN/WLAN HDL/WLAN_Tx_Rx/WLAN_Rx/WLANHDLReceiver/FrameFormatDetectionAndSignalRecovery/storingSignalFields ==
  note: Storing OFDM symbol 6 and 7 until frame format detection is completed
  rst : Inport
  dataIn : Inport  Port=2
  validIn : Inport  Port=3
  symbCount : Inport  Port=4
  formatDetected : Inport  Port=5
  Compare To Constant1 : simulink/Logic and Bit Operations/Compare To Constant  relop=>  const=0  OutDataTypeStr=boolean
  Compare To Constant2 : simulink/Logic and Bit Operations/Compare To Constant  relop===  const=5  OutDataTypeStr=boolean
  Compare To Constant3 : simulink/Logic and Bit Operations/Compare To Constant  relop===  const=6  OutDataTypeStr=boolean
  Constant1 : Constant  OutDataTypeStr=uint8  SampleTime=-1
  Delay : Delay  DelayLength=1
  HDL Counter1 : hdlsllib/Sources/HDL Counter  CountType=Count limited  CountInit=0  CountStep=1  CountMax=2*48-1  CountFromType=Initial value  CountFrom=0  CountResetPort=on  CountLoadPort=off  CountEnbPort=on  CountDirPort=off  CountHitOutputPort=off  CountDataType=Unsigned  CountWordLen=8  CountFracLen=0  CountSampTime=1
  HDL Counter2 : hdlsllib/Sources/HDL Counter  CountType=Count limited  CountInit=0  CountStep=1  CountMax=2*48-1  CountFromType=Initial value  CountFrom=0  CountResetPort=on  CountLoadPort=on  CountEnbPort=on  CountDirPort=off  CountHitOutputPort=off  CountDataType=Unsigned  CountWordLen=8  CountFracLen=0  CountSampTime=1
  Logical Operator : Logic  Operator=OR  AllPortsSameDT=off  OutDataTypeStr=boolean
  Logical Operator1 : Logic  AllPortsSameDT=off  OutDataTypeStr=boolean
  Logical Operator2 : Logic  Operator=OR  AllPortsSameDT=off  OutDataTypeStr=boolean
  Simple Dual Port RAM : hdlsllib/HDL RAMs/Simple Dual Port RAM  ram_size=8
  rd_dout : Outport
  validOut : Outport  Port=2
  wires:
  HDL Counter1/1 -> Simple Dual Port RAM/2
  formatDetected/1 -> HDL Counter2/2, Logical Operator/2
  Constant1/1 -> HDL Counter2/3
  Simple Dual Port RAM/1 -> rd_dout/1
  dataIn/1 -> Simple Dual Port RAM/1
  HDL Counter2/1 -> Simple Dual Port RAM/4, Compare To Constant1/1
  Compare To Constant1/1 -> HDL Counter2/4, Logical Operator/1
  Logical Operator/1 -> Delay/1
  Delay/1 -> validOut/1
  validIn/1 -> Logical Operator1/1
  Logical Operator2/1 -> Logical Operator1/2
  Compare To Constant2/1 -> Logical Operator2/1
  symbCount/1 -> Compare To Constant3/1, Compare To Constant2/1
  Compare To Constant3/1 -> Logical Operator2/2
  Logical Operator1/1 -> HDL Counter1/2, Simple Dual Port RAM/3
  rst/1 -> HDL Counter2/1, HDL Counter1/1

== system soc_WLAN_fpga/WLAN/WLAN HDL/WLAN_Tx_Rx/WLAN_Rx/WLANHDLReceiver/HT_VHTCPEEstAndCorrection/CPECorrector ==
  note: Let Z be the complex CPE estimate and Xbar be the data and X be the corrected data.
      |
      | X = Xbar * conj(Z) * (1/abs(Z))
  dataIn : Inport
  validIn : Inport  Port=2
  estimate : Inport  Port=3
  Complex to Magnitude-Angle HDL Optimized : dsphdlmathfun2/Complex to Magnitude-Angle  NumIterationsSource=Auto  NumIterations=10  OutputFormat=Magnitude  AngleFormat=Normalized  ScaleOutput=on  ScalingMethod=Shift-Add  SimulateUsing=Code generation
  Constant1 : Constant  OutMin=1  OutMax=1  OutDataTypeStr=boolean  SampleTime=1/Fs
  Data Type Conversion : DataTypeConversion  OutDataTypeStr=fixdt(1,14,9)  SaturateOnIntegerOverflow=off  RndMeth=Floor
  Delay : Delay  DelayLength=20
  Delay1 : Delay  DelayLength=20
  Delay{2..4,6..8,10,14..18,22,25,28,36,39} (17 alike) : Delay  InitialCondition=0
  Delay11 : Delay  DelayLength=7  InitialCondition=0
  Delay12 : Delay  DelayLength=7  InitialCondition=0
  Delay5 : Delay  DelayLength=20
  Delay9 : Delay  DelayLength=7  InitialCondition=0
  Math Function : Math  Operator=conj  SignedPower=on  RndMeth=Zero
  Product1 : Product  OutDataTypeStr=Inherit: Same as first input
  Product2 : Product  OutDataTypeStr=Inherit: Same as first input
  Reciprocal : Subsystem  mask{WL=14, FL=9, outWL=26, Mapp=RAM - Based}
      mask prompts: WL "Input Word Length :"; FL "Input Fractional Length :"; outWL "Output Word Length :"; Mapp "Mapping Type:"
      mask init:
      | % Inverse for 18 bit numbers: partitioned into 3+15 bits. 2^3 LUTs with 2^15
      | % combinations will store a total of 2^18 combinations.
      | % As each LUT has 2^15 combinations the data type of output has a maximum
      | % limit of 32 bits (2^20 is a maximum number of bits an LUT can store)
      | 
      | % Non tunable Parameters
      | % FL = 16;
      | % outWL = 31;
      | % WL = 18;
      | % This Parameter is not given for mask
      | LUTAddrWL = WL - 1; % this will implement 2 LUTs
      | 
      | % validate Non tunable parameters
      | % condition for validation: 2^20 bits is the maximum number of bits an LUT can store
      | if LUTAddrWL >= 20   % As 2^20 is the limit
      |     error('invalid LUTAddrWL');
      | end
      | if outWL >= 2^(20-LUTAddrWL)  % 2^(20-LUTAddrWL) is the maximum outWL based on condition for validation
      |     error('invalid outWL')
      | end
      | 
      | % calculate number of LUTs required
      | muxSelectorWL = WL - LUTAddrWL;
      | nLUT = 2^muxSelectorWL;
      | 
      | % Generate all possible RWV inputs using WL and FL
      | allInputRangeSI = -2^(WL-1):2^(WL-1)-1;  % as a stored integer
      | allInputRWV = allInputRangeSI * 2^(-FL);
      | 
      | % define the function for all the RWV input
      | reciprocal = 1./allInputRWV;
      | 
      | % store the function output in LUT
      | allLUTAddr = (0:2^LUTAddrWL-1);
      | LUT = zeros(length(allLUTAddr),nLUT);
      | for i = 0:nLUT-1
      |     LUT(:,i+1) = reciprocal(i*2^LUTAddrWL+1:(i+1)*2^LUTAddrWL);
      | end
      | 
      | % quantize the function with outWL
      | NT = numerictype(fi(LUT(abs(LUT) ~= inf),1,outWL)); % inf and -inf will be quantized with max and min values with NT data type
      | if NT.WordLength < NT. FractionLength
      |     NT.FractionLength = NT.WordLength
      | end
      | LUT = fi(LUT,NT);
      | 
      | paths = find_system([gcb '/Function Impl'],'BlockType','Delay');
      | 
      | for i = 1:length(paths)
      |     if Mapp == 1
      |         hdlset_param(paths{i},'ResetType','default');
      |     else
      |         hdlset_param(paths{i},'ResetType','none');
      |     end
      | end
      mask TypeOptions Mapp: LUT - Based | RAM - Based
      mask DialogControl DescGroupVar Prompt: LUT - Based function
      mask DialogControl DescTextVar Prompt: This block is implemented for complex reciprocal
      mask Display: disp(['Reciprocal\n' get_param(gcb,'Mapp') '\nLatency = 7'])
  Terminator : Terminator
  dataOut : Outport
  validOut : Outport  Port=2
  wires:
  Delay7/1 -> Delay17/1
  Complex to Magnitude-Angle HDL Optimized/1 -> Delay10/1
  Constant1/1 -> Complex to Magnitude-Angle HDL Optimized/2
  Product1/1 -> Delay39/1
  Reciprocal/1(dataOut) -> Delay3/1
  estimate/1 -> Complex to Magnitude-Angle HDL Optimized/1, Delay1/1
  Delay36/1 -> Product2/1
  Delay1/1 -> Delay25/1
  Delay25/1 -> Delay9/1
  Math Function/1 -> Delay28/1
  Delay28/1 -> Product2/2
  Delay16/1 -> Delay18/1
  Delay22/1 -> validOut/1
  Delay39/1 -> dataOut/1
  Product2/1 -> Delay4/1
  Delay14/1 -> Delay16/1
  Delay2/1 -> Delay12/1
  Delay5/1 -> Delay2/1
  validIn/1 -> Delay5/1
  dataIn/1 -> Delay/1
  Delay/1 -> Delay8/1
  Delay8/1 -> Delay11/1
  Delay4/1 -> Delay15/1
  Delay6/1 -> Terminator/1
  Delay9/1 -> Math Function/1
  Delay11/1 -> Delay36/1
  Delay12/1 -> Delay14/1
  Delay15/1 -> Product1/1
  Delay17/1 -> Product1/2
  Delay18/1 -> Delay22/1
  Delay3/1 -> Delay7/1
  Delay10/1 -> Data Type Conversion/1
  Data Type Conversion/1 -> Reciprocal/1(dataIn)
  Complex to Magnitude-Angle HDL Optimized/2 -> Delay6/1

== system soc_WLAN_fpga/WLAN/WLAN HDL/WLAN_Tx_Rx/WLAN_Rx/WLANHDLReceiver/HT_VHTCPEEstAndCorrection/CPEEstimator ==
  note: delay the adder output till the end of Symbol
      | delay value = Maximum Used subcarrier-
      |  Last pilot Subcarrier position
  note: add the pilots; reset the pilots for every Symbol
  note: Multiply the Equalizer Output with reference pilots
  dataOut : Inport
  pilotScValid : Inport  Port=2
  SymbolEndInd : Inport  Port=3
  polarity : Inport  Port=4
  vhtSigB : Inport  Port=5
  rst : Inport  Port=6
  Add : Sum  OutDataTypeStr=Inherit: Same as first input
  Constant : Constant  Value=complex(0,0)  OutDataTypeStr=Inherit: Inherit via back propagation  SampleTime=-1
  Constant1 : Constant  Value=0  OutDataTypeStr=Inherit: Inherit via back propagation  SampleTime=-1
  Data Type Conversion : DataTypeConversion  OutDataTypeStr=fixdt(1,16,10)  SaturateOnIntegerOverflow=off  RndMeth=Floor
  Delay : Delay  DelayLength=1  ExternalReset=Level
      settings: InputPortMap=u0,r5
  Delay1 : Delay  DelayLength=numPilots-1
  Delay{2..6} (5 alike) : Delay  DelayLength=1  InitialCondition=0  UseCircularBuffer=on
  Product : Product  OutDataTypeStr=Inherit: Same as first input
  Product1 : Product  OutDataTypeStr=Inherit: Same as first input
  Real-Imag to Complex : RealImagToComplex
  RefrenceSignalGen : Subsystem
  Switch : Switch  Criteria=u2 > Threshold  SaturateOnIntegerOverflow=off  InputSameDT=off
  sampleAndHold : MATLAB Function  TreatAsAtomicUnit=on
  x : Outport
  wires:
  Switch/1 -> Data Type Conversion/1
  Constant/1 -> Switch/3
  Constant1/1 -> Real-Imag to Complex/2
  Delay/1 -> Add/2
  Add/1 -> Delay1/1, Delay/1
  Product/1 -> Switch/1
  RefrenceSignalGen/1(RefPilotsOut) -> Real-Imag to Complex/1
  SymbolEndInd/1 -> Delay5/1
  dataOut/1 -> Delay6/1
  Product1/1 -> Product/2
  Delay1/1 -> sampleAndHold/1(x)
  Real-Imag to Complex/1 -> Product1/1
  polarity/1 -> Delay3/1
  pilotScValid/1 -> Delay4/1, RefrenceSignalGen/1(loadIn)
  vhtSigB/1 -> RefrenceSignalGen/2(vhtSigB)
  rst/1 -> sampleAndHold/3(rst), RefrenceSignalGen/3(rst)
  Data Type Conversion/1 -> Add/1
  sampleAndHold/1(y) -> Delay2/1
  Delay2/1 -> x/1
  Delay3/1 -> Product1/2
  Delay4/1 -> Switch/2
  Delay5/1 -> sampleAndHold/2(enb), Delay/2
  Delay6/1 -> Product/1

== system soc_WLAN_fpga/WLAN/WLAN HDL/WLAN_Tx_Rx/WLAN_Rx/WLANHDLReceiver/HT_VHTCPEEstAndCorrection/PilotSubCarrierSelector ==
  note: Pilot Subcarriers are stored in LUT. Note that subcarriers positions other than pilots subcarriers positions are stored with Max Value outside the range of Subcarriers
  note: Count Used Subcarriers and generate pulse at the end of the Symbol
  note: Pilot Subcarriers are selected by comparing with counter value and LUT output
  validIn : Inport
  rst : Inport  Port=2
  1-D Lookup Table : Lookup_n-D  NumberOfTableDimensions=1  BreakpointsForDimension1=[0:numSCS_HT-1]  IndexSearchMethod=Evenly spaced points  Table=HTLUTPilots.'  ExtrapMethod=Clip  UseLastTableValue=on  InternalRulePriority=Speed  OutDataTypeStr=uint8  RndMeth=Simplest
  Compare To Zero : simulink/Logic and Bit Operations/Compare To Zero  relop===  OutDataTypeStr=boolean
  Delay{,1..3} (4 alike) : Delay  DelayLength=1  InitialCondition=0  UseCircularBuffer=on
  HDL Counter : hdlsllib/Sources/HDL Counter  CountType=Count limited  CountInit=0  CountStep=1  CountMax=numSCS_HT-1  CountFromType=Initial value  CountFrom=0  CountResetPort=on  CountLoadPort=off  CountEnbPort=on  CountDirPort=off  CountHitOutputPort=on  CountDataType=Unsigned  CountWordLen=maxNsdCounterWL  CountFracLen=0  CountSampTime=1
  Logical Operator : Logic  AllPortsSameDT=off  OutDataTypeStr=boolean
  Relational Operator : RelationalOperator  Operator===  OutDataTypeStr=boolean  RndMeth=Simplest  InputSameDT=off
  pilotScValidOut : Outport  VectorParamsAs1DForOutWhenUnconnected=off
  SymbEndInd : Outport  Port=2  VectorParamsAs1DForOutWhenUnconnected=off
  SymbStart : Outport  Port=3  VectorParamsAs1DForOutWhenUnconnected=off
  wires:
  validIn/1 -> Delay3/1, HDL Counter/2
  HDL Counter/2 -> Delay2/1
  Logical Operator/1 -> SymbStart/1
  Relational Operator/1 -> pilotScValidOut/1
  1-D Lookup Table/1 -> Delay/1
  HDL Counter/1 -> 1-D Lookup Table/1, Delay1/1
  Compare To Zero/1 -> Logical Operator/1
  rst/1 -> HDL Counter/1
  Delay/1 -> Relational Operator/1
  Delay1/1 -> Relational Operator/2, Compare To Zero/1
  Delay2/1 -> SymbEndInd/1
  Delay3/1 -> Logical Operator/2

== system soc_WLAN_fpga/WLAN/WLAN HDL/WLAN_Tx_Rx/WLAN_Rx/WLANHDLReceiver/HT_VHTCPEEstAndCorrection/PolarityGenerator ==
  note: Choose polarity 1 for VHT Sig B
  note: Choose ZStart based on Format detected
  enb : Inport
  formatDetected : Inport  Port=2
  VHTSigB : Inport  Port=3
  rst : Inport  Port=4
  1-D Lookup Table : Lookup_n-D  NumberOfTableDimensions=1  BreakpointsForDimension1=0:126  BreakpointsForDimension1FirstPoint=0  IndexSearchMethod=Evenly spaced points  Table=pnSeq  TableDataTypeStr=fixdt(1,2,0)  ExtrapMethod=Clip  UseLastTableValue=on  InternalRulePriority=Speed  OutDataTypeStr=fixdt(1,2,0)  RndMeth=Simplest
  Compare To Zero : simulink/Logic and Bit Operations/Compare To Zero  relop===  OutDataTypeStr=boolean
  Constant : Constant  Value=fi(1,1,2,0)  SampleTime=-1
  Constant1 : Constant  Value=3  OutDataTypeStr=fixdt(0,7,0)  SampleTime=-1
  Constant2 : Constant  Value=4  OutDataTypeStr=fixdt(0,7,0)  SampleTime=-1
  Delay : Delay  DelayLength=1  InitialCondition=0  UseCircularBuffer=on
  Delay1 : Delay  DelayLength=1  InitialCondition=0  UseCircularBuffer=on
  HDL Counter : hdlsllib/Sources/HDL Counter  CountType=Count limited  CountInit=0  CountStep=1  CountMax=126  CountFromType=Initial value  CountFrom=0  CountResetPort=on  CountLoadPort=on  CountEnbPort=on  CountDirPort=off  CountHitOutputPort=off  CountDataType=Unsigned  CountWordLen=7  CountFracLen=0  CountSampTime=1
  HDL Counter1 : hdlsllib/Sources/HDL Counter  CountType=Count limited  CountInit=0  CountStep=1  CountMax=65535  CountFromType=Initial value  CountFrom=0  CountResetPort=on  CountLoadPort=off  CountEnbPort=on  CountDirPort=off  CountHitOutputPort=off  CountDataType=Unsigned  CountWordLen=16  CountFracLen=0  CountSampTime=1
  Logical Operator : Logic  AllPortsSameDT=off  OutDataTypeStr=boolean
  Logical Operator1 : Logic  AllPortsSameDT=off  OutDataTypeStr=boolean
  Logical Operator2 : Logic  Operator=NOT  AllPortsSameDT=off  OutDataTypeStr=boolean
  Switch : Switch  Criteria=u2 > Threshold  Threshold=1  SaturateOnIntegerOverflow=off  InputSameDT=off
  Switch1 : Switch  Criteria=u2 ~= 0  SaturateOnIntegerOverflow=off  InputSameDT=off
  polarity : Outport
  vhtSigB : Outport  Port=2
  wires:
  Logical Operator1/1 -> HDL Counter/4, Logical Operator/2, HDL Counter1/2
  HDL Counter/1 -> 1-D Lookup Table/1
  Logical Operator/1 -> HDL Counter/2
  Constant1/1 -> Switch/3
  HDL Counter1/1 -> Compare To Zero/1
  Compare To Zero/1 -> Logical Operator/1
  Constant2/1 -> Switch/1
  formatDetected/1 -> Switch/2
  1-D Lookup Table/1 -> Delay/1
  VHTSigB/1 -> Delay1/1, Logical Operator2/1
  Logical Operator2/1 -> Logical Operator1/2
  enb/1 -> Logical Operator1/1
  Switch1/1 -> polarity/1
  Switch/1 -> HDL Counter/3
  rst/1 -> HDL Counter/1, HDL Counter1/1
  Delay/1 -> Switch1/3
  Delay1/1 -> Switch1/2, vhtSigB/1
  Constant/1 -> Switch1/1
